simulink model "absbrake_expanded"  (R2017a)
settings: Solver=ode45  StartTime=0.0  StopTime=25  MaxStep=.01  RelTol=1e-3  AbsTol=1e-6
PreLoadFcn:
  | % Load initialization data
  | 
  | sldemo_absdata;
StopFcn:
  | %if exist ('sldemo_absbrake_output')
  | %  sldemo_absbrakeplots;
  | %end
model workspace: external: MAT-File absbrake_expanded_params.mat (data not in the file)
undefined symbols (not defined in the file or in its folder): ctrl, g, I, m, mu, PBmax, Rr, slip, TB, v0
CloseFcn:
  | % Close the plots that are still open
  | %h = findobj(0, 'Name', 'ABS Speeds');
  | %if ~isempty(h),
  | %  close(h);
  | %end;
  | 
  | %h = findobj(0, 'Name', 'ABS Slip');
  | %if ~isempty(h),
  |  % close(h);
  | %end;
  | 
  | % Clear initial conditions data to avoid cluttering the workspace
  | 
  | %clear g v0 Rr Kf m PBmax TB I slip mu ctrl h;
Description:
  | Modeling an Anti-Lock Braking System (ABS)
  | 
  | *Summary*
  | 
  | This example describes a simple model for an Anti-Lock Braking System
  | (ABS). The model simulates the dynamic behavior of a vehicle
  | under hard braking conditions. The model represents a single wheel, which
  | may be replicated a number of times to create a model for a multi-wheel
  | vehicle.
  | 
  | This model uses the signal logging feature in Simulink(R). You log signals to the
  | MATLAB(R) workspace where you can analyze and view them. You can view
  | the code in sldemo_absbrakeplots.m to see how this is done.
  | 
  | In this model, the wheel speed is calculated in a separate component
  | named sldemo_wheelspeed_absbrake.
  | This component is then referenced using a Model block.  Note that both the
  | top model and the referenced model use a variable step solver, so Simulink
  | will track zero-crossings in the referenced model.
settings Model: FPTRunName=Active  ExtModeTrigMode=oneshot  ExtModeArmWhenConnect=off  ExtModeAutoUpdateStatusClock=off  Creator=The MathWorks, Inc.  LastModifiedBy=nikhil
settings DataIOCC: SaveFormat=Array  SaveOutput=off  SaveTime=off  TimeSaveName=time  SignalLoggingName=sldemo_absbrake_output
settings OptimizationCC: DefaultParameterBehavior=Inlined  InlineInvariantSignals=on  ExpressionDepthLimit=2147483647  InitFltsAndDblsToZero=on  LifeSpan=inf  BufferReusableBoundary=off
settings DebuggingCC: SaveWithParameterizedLinksMsg=none  UnderspecifiedInitializationDetection=Classic  MergeDetectMultiDrivingBlocksExec=none  MultiTaskDSMMsg=warning  SigSpecEnsureSampleTimeMsg=none  IntegerOverflowMsg=none  FcnCallInpInsideContextMsg=warning  BusObjectLabelMismatch=none  AllowSymbolicDim=off  StateNameClashWarn=warning  SFUnexpectedBacktrackingDiag=warning  SFNoUnconditionalDefaultTransitionDiag=warning  SFExecutionAtInitializationDiag=none  IntegerSaturationMsg=none
settings HardwareCC: ProdBitPerPointer=32  ProdBitPerSizeT=32  ProdBitPerPtrDiffT=32  ProdLargestAtomicFloat=None  ProdIntDivRoundTo=Undefined  ProdEndianess=Unspecified  ProdWordSize=32  ProdHWDeviceType=32-bit Generic  TargetBitPerLong=64  TargetBitPerPointer=64  TargetBitPerSizeT=64  TargetBitPerPtrDiffT=64  TargetLongLongMode=on  TargetIntDivRoundTo=Zero  TargetEndianess=LittleEndian  TargetWordSize=64  TargetHWDeviceType=MATLAB Host
settings ModelReferenceCC: UpdateModelReferenceTargets=IfOutOfDate  PropagateSignalLabelsOutOfModel=off
settings GRTTargetCC: TargetLangStandard=C89/C90 (ANSI)  GeneratePreprocessorConditionals=Disable all
settings ConfigComp: CovMetricSettings=dw  CovHtmlReporting=on  CovSaveCumulativeToWorkspaceVar=on  CovSaveSingleToWorkspaceVar=on  CovExternalEMLEnable=off  CovSFcnEnable=off

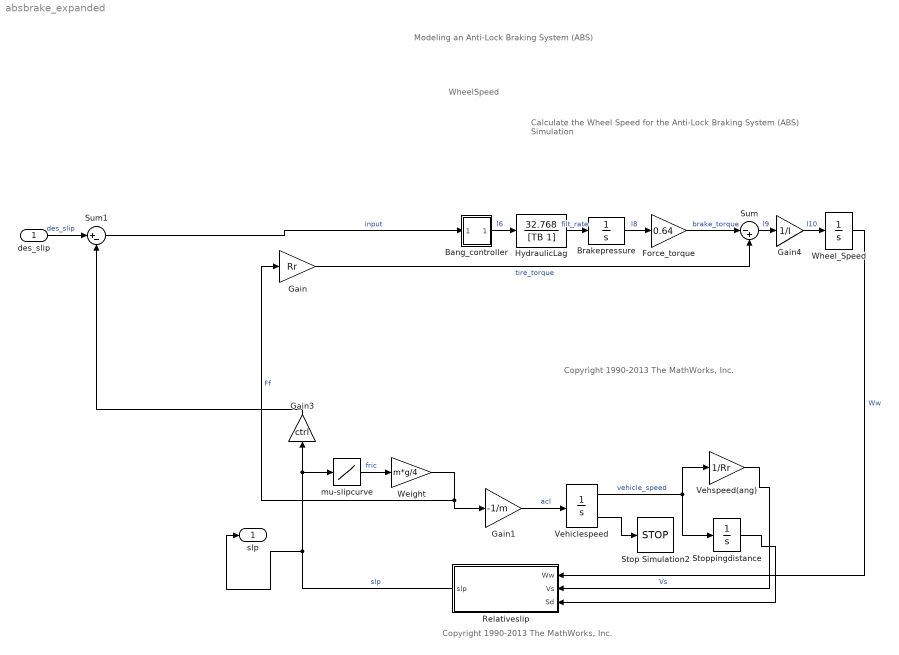
== system absbrake_expanded ==
  note: WheelSpeed
  note: Modeling an Anti-Lock Braking System (ABS)
  note: Copyright 1990-2013 The MathWorks, Inc.
  note: Calculate the Wheel Speed for the
      | Anti-Lock Braking System (ABS) Simulation
  note: Copyright 1990-2013 The MathWorks, Inc.
  des_slip : Inport
  Bang_controller : Subsystem  TreatAsAtomicUnit=on
  Brakepressure : Integrator  LimitOutput=on  UpperSaturationLimit=PBmax  LowerSaturationLimit=0
  Force_torque : Gain  Gain=0.64  SaturateOnIntegerOverflow=on  OutDataTypeStr=Inherit: Same as input  ParamDataTypeStr=Inherit: Same as input
  Gain : Gain  Gain=Rr  SaturateOnIntegerOverflow=on  OutDataTypeStr=Inherit: Same as input  ParamDataTypeStr=Inherit: Same as input
  Gain1 : Gain  Gain=-1/m  SaturateOnIntegerOverflow=on  OutDataTypeStr=Inherit: Same as input  ParamDataTypeStr=Inherit: Same as input
  Gain3 : Gain  Gain=ctrl  SaturateOnIntegerOverflow=on  OutDataTypeStr=Inherit: Same as input  ParamDataTypeStr=Inherit: Same as input
  Gain4 : Gain  Gain=1/I  SaturateOnIntegerOverflow=on  OutDataTypeStr=Inherit: Same as input  ParamDataTypeStr=Inherit: Same as input
  HydraulicLag : TransferFcn  Numerator=32.768  Denominator=[TB 1]
  Relativeslip : Subsystem  TreatAsAtomicUnit=on
  Stop Simulation2 : Stop
  Stoppingdistance : Integrator  UpperSaturationLimit=1000  LowerSaturationLimit=0
  Sum : Sum  Inputs=|-+  SaturateOnIntegerOverflow=on  InputSameDT=on  OutDataTypeStr=Inherit: Same as first input
  Sum1 : Sum  Inputs=|+-  SaturateOnIntegerOverflow=on  InputSameDT=on  OutDataTypeStr=Inherit: Same as first input
  Vehiclespeed : Integrator  InitialCondition=v0  LimitOutput=on  UpperSaturationLimit=1000  LowerSaturationLimit=0  ShowSaturationPort=on
  Vehspeed(ang) : Gain  Gain=1/Rr  SaturateOnIntegerOverflow=on  OutDataTypeStr=Inherit: Same as input  ParamDataTypeStr=Inherit: Same as input
  Weight : Gain  Gain=m*g/4  SaturateOnIntegerOverflow=on  OutDataTypeStr=Inherit: Same as input  ParamDataTypeStr=Inherit: Same as input
  Wheel_Speed : Integrator  InitialCondition=v0/Rr  LimitOutput=on  UpperSaturationLimit=1000  LowerSaturationLimit=0
  mu-slipcurve : Lookup_n-D  NumberOfTableDimensions=1  BreakpointsForDimension1=slip  Table=mu  SaturateOnIntegerOverflow=on  InputSameDT=on
  slp : Outport
  wires:
  Vehspeed(ang)/1 -> Relativeslip/2(Vs)  "Vs"
  Relativeslip/1(slp) -> slp/1, mu-slipcurve/1, Gain3/1  "slp"
  Stoppingdistance/1 -> Relativeslip/3(Sd)
  Gain1/1 -> Vehiclespeed/1  "acl"
  Vehiclespeed/2 -> Stop Simulation2/1
  Vehiclespeed/1 -> Stoppingdistance/1, Vehspeed(ang)/1  "vehicle_speed"
  mu-slipcurve/1 -> Weight/1  "fric"
  Weight/1 -> Gain1/1, Gain/1  "Ff"
  Gain3/1 -> Sum1/2
  des_slip/1 -> Sum1/1  "des_slip"
  Sum1/1 -> Bang_controller/1(in_1)  "input"
  Gain/1 -> Sum/2  "tire_torque"
  Brakepressure/1 -> Force_torque/1  "l8"
  Gain4/1 -> Wheel_Speed/1  "l10"
  Wheel_Speed/1 -> Relativeslip/1(Ww)  "Ww"
  Sum/1 -> Gain4/1  "l9"
  Force_torque/1 -> Sum/1  "brake_torque"
  Bang_controller/1(out_1) -> HydraulicLag/1  "l6"
  HydraulicLag/1 -> Brakepressure/1  "filt_rate"

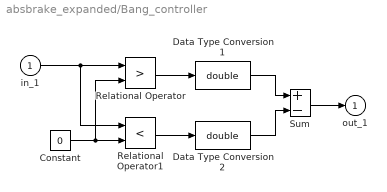
== system absbrake_expanded/Bang_controller ==
  in_1 : Inport
  Constant : Constant  Value=0
  Data Type Conversion1 : DataTypeConversion  OutDataTypeStr=double  SaturateOnIntegerOverflow=on  RndMeth=Zero
  Data Type Conversion2 : DataTypeConversion  OutDataTypeStr=double  SaturateOnIntegerOverflow=on  RndMeth=Zero
  Relational Operator : RelationalOperator  Operator=>  OutDataTypeStr=boolean  RndMeth=Nearest  InputSameDT=on
  Relational Operator1 : RelationalOperator  Operator=<  OutDataTypeStr=boolean  RndMeth=Nearest  InputSameDT=on
  Sum : Sum  Inputs=+-  SaturateOnIntegerOverflow=on  InputSameDT=on  OutDataTypeStr=Inherit: Same as first input
  out_1 : Outport  InitialOutput=0
  wires:
  Data Type Conversion2/1 -> Sum/2
  Data Type Conversion1/1 -> Sum/1
  Sum/1 -> out_1/1
  Relational Operator/1 -> Data Type Conversion1/1
  Relational Operator1/1 -> Data Type Conversion2/1
  Constant/1 -> Relational Operator/2, Relational Operator1/2
  in_1/1 -> Relational Operator1/1, Relational Operator/1

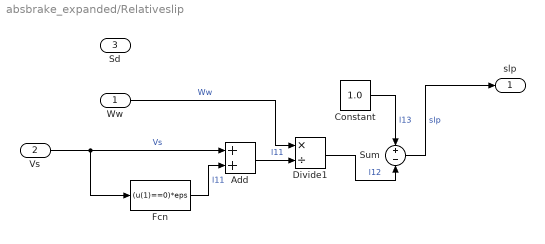
== system absbrake_expanded/Relativeslip ==
  Ww : Inport
  Vs : Inport  Port=2
  Sd : Inport  Port=3
  Add : Sum
  Constant : Constant  Value=1.0
  Divide1 : Product  Inputs=*/
  Fcn : Fcn  Expr=(u(1)==0)*eps
  Sum : Sum  Inputs=+|-
  slp : Outport
  wires:
  Sum/1 -> slp/1  "slp"
  Ww/1 -> Divide1/1  "Ww"
  Vs/1 -> Fcn/1, Add/1  "Vs"
  Fcn/1 -> Add/2  "l11"
  Add/1 -> Divide1/2  "l11"
  Constant/1 -> Sum/1  "l13"
  Divide1/1 -> Sum/2  "l12"
